simulink model "sm_pick_and_place_robot"  (R2021b)
settings: Solver=ode3  StartTime=0.0  StopTime=1.5  FixedStep=dt_solver  RelTol=1e-3  AbsTol=1e-3
model workspace (MAT data in the model file):
  dt_planner = 0.001
  dt_solver = 0.0002
undefined symbols (not defined in the file or in its folder): DiscIntNeverNeededParam, entire, Marker1, Marker2, Marker3, Marker4, point1, point2, point3, X, Y, Z
libraries: sm_lib x32, nesl_utility x17, sm_delta_robot_lib x1
(part 1 of 2)
CloseFcn:
  | clear sm_pick_and_place_robot_ik
  | clear sm_pick_and_place_robot_fk
Description:
  | Pick and Place Robot with Forward and Inverse Kinematics
settings Model: Creator=The MathWorks, Inc.  LastModifiedBy=The MathWorks, Inc.
settings SolverCC: AlgebraicLoopSolver=TrustRegion
settings DataIOCC: ReturnWorkspaceOutputs=off
settings DebuggingCC: SFMachineParentedDataDiag=warning
settings SimscapeCC: SimscapeLogType=all  SimscapeLogSimulationStatistics=on  SimscapeLogName=simlog_sm_pick_and_place_robot  SimscapeLogDataHistory=10000
settings ExplorerConfigSet: InternalSimMechanicsExplorerSettings="<ExplorerConfiguration><canonicalview>default</canonicalview><AnimationSetting><BasePlaybackSpeed>1.0</BasePlaybackSpeed><PlaybackSpeedFactor>1.0</PlaybackSpeedFactor></AnimationSetting><TilePanel><TileInfo><Tiles Columns=\"2\" Count=\"3\" Rows=\"2\"><Column Weight=\"0.5\"/><Column Weight=\"0.5\"/><Row Weight=\"0.3038\"/><Row Weight=\"0.6962\"/><Tile Height=\"2\" Width=\"1\" X=\"0\" Y=\"0\"/><Tile Height=\"1\" Width=\"1\" X=\"1\" Y=\"0\"/><Tile Height=\"1\" Width=\"1\" X=\"1\" Y=\"1\"/></Tiles></TileInfo><SceneInfo><SceneViewer><BGColor><R>0.60000002384185791</R><G>0.60000002384185791</G><B>0.60000002384185791</B></BGColor><Camera><DoPerspective>off</DoPerspective><Position><X>0.674555883500480347</X><Y>-0.674555883500480902</Y><Z>0.921885249943208973</Z></Position><Center><X>0.0060149771328419227</X><Y>-0.00601497713284246394</Y><Z>0.253344343575570674</Z></Center><Up><X>-0.408248290463863073</X><Y>0.408248290463863073</Y><Z>0.816496580927726145</Z></Up><ViewLimDist>1</ViewLimDist><YLim>0.43506960332393646</YLim><XLim>0.392966093324845833</XLim></Camera></SceneViewer><SceneViewer><BGColor><R>0.60000002384185791</R><G>0.60000002384185791</G><B>0.60000002384185791</B></BGColor><Camera><DoPerspective>off</DoPerspective><Position><X>-0.000385309004919674389</X><Y>-1.33915517216324798</Y><Z>0.0518624305243804845</Z></Position><Center><X>-0.000385309004919674389</X><Y>0.0454699993133544367</Y><Z>0.0518624305243804845</Z></Center><Up><X>0</X><Y>-0</Y><Z>1</Z></Up><ViewLimDist>1</ViewLimDist><YLim>0.0894075615531887413</YLim><XLim>0.282074560393158813</XLim></Camera></SceneViewer><SceneViewer><BGColor><R>0.60000002384185791</R><G>0.60000002384185791</G><B>0.60000002384185791</B></BGColor><Camera><DoPerspective>on</DoPerspective><Position><X>-1.13755508710961844e-18</X><Y>-8.63362207815730793e-18</Y><Z>0.589999999999999969</Z></Position><Center><X>-1.13755508710961844e-18</X><Y>-8.63362207815730793e-18</Y><Z>-0.410000000000000031</Z></Center><Up><X>0</X><Y>1</Y><Z>0</Z></Up><ViewLimDist>1</ViewLimDist><YLim>0.466307658154998583</YLim><XLim>0.621743544206664778</XLim></Camera></SceneViewer></SceneInfo></TilePanel><MechEditorPanel><Cameras><Camera><Id>Camera1</Id><Value><Name>CameraView</Name><NativeCamera><PositionTrackingFeature>Delta_Robot.Camera_Frame</PositionTrackingFeature><CenterTrackingFeature>Delta_Robot.Camera_Frame</CenterTrackingFeature><UpVectorTrackingFeature>Delta_Robot.Camera_Frame</UpVectorTrackingFeature><CenterTrackingOrigin>off</CenterTrackingOrigin><CenterTrackingDirection>+Z</CenterTrackingDirection><UpVectorTrackingDirection>-Y</UpVectorTrackingDirection></NativeCamera></Value></Camera></Cameras><GfxPanelCameraMap><MapElement CameraMLId=\"Camera1\" GfxPanelIndex=\"2\"/></GfxPanelCameraMap><VideoCreator><PlaybackSpeedRatio>1.0</PlaybackSpeedRatio><FrameRate>30</FrameRate><VideoFormat>Motion JPEG AVI</VideoFormat><FrameSize>auto</FrameSize></VideoCreator></MechEditorPanel></ExplorerConfiguration>"

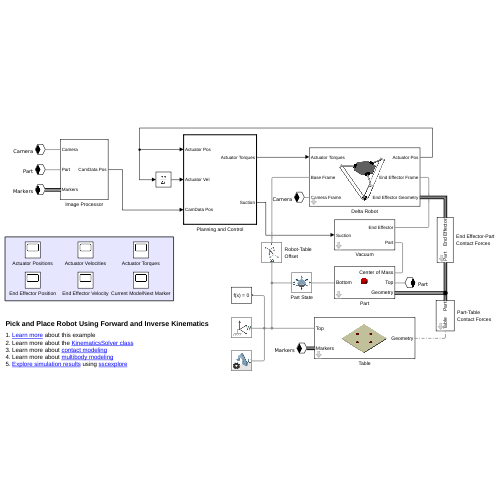
[thumbnail: Simulink's stored preview of the top-level diagram]
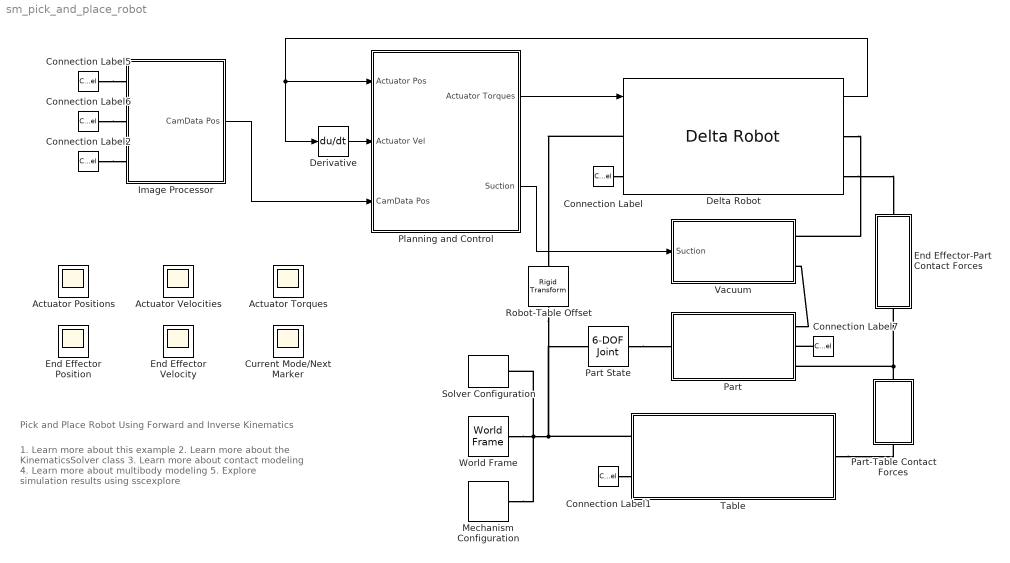
== system sm_pick_and_place_robot ==
  note: Pick and Place Robot Using Forward and Inverse Kinematics
  note: 1. Learn more about this example
      | 2. Learn more about the KinematicsSolver class
      | 3. Learn more about contact modeling
      | 4. Learn more about multibody modeling
      | 5. Explore simulation results using sscexplore
  Actuator Positions : Scope
      settings: Floating=on
  Actuator Torques : Scope
      settings: Floating=on
  Actuator Velocities : Scope
      settings: Floating=on
  Connection Label : ConnectionLabel  Label=Camera
  Connection Label1 : ConnectionLabel  Label=Markers
  Connection Label2 : ConnectionLabel  Label=Markers
  Connection Label5 : ConnectionLabel  Label=Camera
  Connection Label6 : ConnectionLabel  Label=Part
  Connection Label7 : ConnectionLabel  Label=Part
  Current Mode/Next Marker : Scope
      settings: Floating=on
  Delta Robot : sm_delta_robot_lib/Delta Robot  Rtop=0.15  Rbot=0.03  L1=0.2  R1=0.01  L2=0.5  L3=0.07  R2=0.005  eeL=0.03  eeR=0.01  th0=[10; 10; 10]  thd0=[0 0 0]  mask(Delta Robot){}
      mask init:
      | clear delta_robot_kf delta_robot_ik
      settings: SourceProductBaseCode=MS
  Derivative : Derivative  CoefficientInTFapproximation=dt_planner
  End Effector Position : Scope
      settings: Floating=on
  End Effector Velocity : Scope
      settings: Floating=on
  End Effector-Part Contact Forces : Subsystem  mask(End Effector-Part Contact Forces){k=1e6, b=10, mus=0.4, muk=0.4}
      mask prompts: k "Stiffness (N/m)"; b "Damping (N/(m/s))"; mus "Coefficient of Static Friction"; muk "Coefficient of Dynamic Friction"
      mask help: This block models the contact forces between the end effector and the part. The entire cylindrical part geometry is used, but the end effector geometry corresponds to the three contact points around the tip.
  Image Processor : Subsystem
  Mechanism Configuration : sm_lib/Utilities/Mechanism Configuration  UniformGravity=Constant  GravityVector=[0 0 -9.80665]  GravityUnits=m/s^2  LinearizationDelta=0.001  JointModeTransitionNonlinearIterations=2
  Part : Subsystem  mask(Part){R=0.02, H=0.02}
      mask prompts: R "Radius (m)"; H "Height (m)"
      mask help: This block models a cylindrical part. Frames at the center of the bottom face, center of the top face, and center of mass are exposed as ports. A Simscape Bus with geometry signals is also exposed. The bus includes the geometry of the entire part as well as the geometries of three evenly spaced points located around the edge of the bottom face of the cylinder.
      mask DialogControl ParameterGroupVar Prompt: Geometry
      mask Display: image(fullfile(matlabroot,'toolbox','physmod','sm','smdemos','pick_and_place_robot','images','sm_pick_and_place_robot_part.png'));
  Part State : sm_lib/Joints/6-DOF Joint  JointMode=Normal  SenseConstraintForce=off  SenseConstraintForceX=off  SenseConstraintForceY=off  SenseConstraintForceZ=off  SenseConstraintTorque=off  SenseConstraintTorqueX=off  SenseConstraintTorqueY=off  SenseConstraintTorqueZ=off  SenseTotalForce=off  SenseTotalForceX=off  SenseTotalForceY=off  SenseTotalForceZ=off  SenseTotalTorque=off  SenseTotalTorqueX=off  SenseTotalTorqueY=off  SenseTotalTorqueZ=off  CompositeWrenchDir=FollowerOnBase  CompositeWrenchFrame=BaseFrame  PxEquilibriumPosition=0  PxEquilibriumPositionUnits=m  PxSpringStiffness=0  PxSpringStiffnessUnits=N/m  PxDampingCoefficient=0  PxDampingCoefficientUnits=N/(m/s)  PxTorqueActuationMode=NoTorque  PxMotionActuationMode=ComputedMotion  PxSensePosition=off  PxSenseVelocity=off  PxSenseAcceleration=off  PxSenseTorqueForce=off  PxSenseLowerLimitTorqueForce=off  PxSenseUpperLimitTorqueForce=off  PxLowerLimitSpecify=off  PxLowerLimitBound=-1  PxLowerLimitBoundUnits=m  PxLowerLimitStiffness=1e6  PxLowerLimitStiffnessUnits=N/m  PxLowerLimitDamping=1e3  PxLowerLimitDampingUnits=N/(m/s)  PxLowerLimitTransitionRegionWidth=1e-4  PxLowerLimitTransitionRegionWidthUnits=m  PxUpperLimitSpecify=off  PxUpperLimitBound=1  PxUpperLimitBoundUnits=m  PxUpperLimitStiffness=1e6  PxUpperLimitStiffnessUnits=N/m  PxUpperLimitDamping=1e3  PxUpperLimitDampingUnits=N/(m/s)  PxUpperLimitTransitionRegionWidth=1e-4  PxUpperLimitTransitionRegionWidthUnits=m  PxPositionTargetSpecify=off  PxPositionTargetPriority=High  PxPositionTargetValue=0  PxPositionTargetValueUnits=m  PxVelocityTargetSpecify=off  PxVelocityTargetPriority=High  PxVelocityTargetValue=0  PxVelocityTargetValueUnits=m/s  PyEquilibriumPosition=0  PyEquilibriumPositionUnits=m  PySpringStiffness=0  PySpringStiffnessUnits=N/m  PyDampingCoefficient=0  PyDampingCoefficientUnits=N/(m/s)  PyTorqueActuationMode=NoTorque  PyMotionActuationMode=ComputedMotion  PySensePosition=off  PySenseVelocity=off  PySenseAcceleration=off  PySenseTorqueForce=off  PySenseLowerLimitTorqueForce=off  PySenseUpperLimitTorqueForce=off  PyLowerLimitSpecify=off  PyLowerLimitBound=-1  PyLowerLimitBoundUnits=m  PyLowerLimitStiffness=1e6  PyLowerLimitStiffnessUnits=N/m  PyLowerLimitDamping=1e3  PyLowerLimitDampingUnits=N/(m/s)  PyLowerLimitTransitionRegionWidth=1e-4  PyLowerLimitTransitionRegionWidthUnits=m  PyUpperLimitSpecify=off  PyUpperLimitBound=1  PyUpperLimitBoundUnits=m  PyUpperLimitStiffness=1e6  PyUpperLimitStiffnessUnits=N/m  PyUpperLimitDamping=1e3  PyUpperLimitDampingUnits=N/(m/s)  PyUpperLimitTransitionRegionWidth=1e-4  PyUpperLimitTransitionRegionWidthUnits=m  PyPositionTargetSpecify=off  PyPositionTargetPriority=High  PyPositionTargetValue=0  PyPositionTargetValueUnits=m  PyVelocityTargetSpecify=off  PyVelocityTargetPriority=High  PyVelocityTargetValue=0  PyVelocityTargetValueUnits=m/s  PzEquilibriumPosition=0  PzEquilibriumPositionUnits=m  PzSpringStiffness=0  PzSpringStiffnessUnits=N/m  PzDampingCoefficient=0  PzDampingCoefficientUnits=N/(m/s)  PzTorqueActuationMode=NoTorque  PzMotionActuationMode=ComputedMotion  PzSensePosition=off  PzSenseVelocity=off  PzSenseAcceleration=off  PzSenseTorqueForce=off  PzSenseLowerLimitTorqueForce=off  PzSenseUpperLimitTorqueForce=off  PzLowerLimitSpecify=off  PzLowerLimitBound=-1  PzLowerLimitBoundUnits=m  PzLowerLimitStiffness=1e6  PzLowerLimitStiffnessUnits=N/m  PzLowerLimitDamping=1e3  PzLowerLimitDampingUnits=N/(m/s)  PzLowerLimitTransitionRegionWidth=1e-4  PzLowerLimitTransitionRegionWidthUnits=m  PzUpperLimitSpecify=off  PzUpperLimitBound=1  PzUpperLimitBoundUnits=m  PzUpperLimitStiffness=1e6  PzUpperLimitStiffnessUnits=N/m  PzUpperLimitDamping=1e3  PzUpperLimitDampingUnits=N/(m/s)  PzUpperLimitTransitionRegionWidth=1e-4  PzUpperLimitTransitionRegionWidthUnits=m  PzPositionTargetSpecify=on  PzPositionTargetPriority=High  PzPositionTargetValue=0  PzPositionTargetValueUnits=m  PzVelocityTargetSpecify=off  PzVelocityTargetPriority=High  PzVelocityTargetValue=0  PzVelocityTargetValueUnits=m/s  SphDefPosRotationMethod=None  SphDefPosRotationAngleUnits=deg  SphDefPosRotationStandardAxis=+Z  SphDefPosRotationAngle=0.0  SphDefPosRotationArbitraryAxis=[0 0 1]  SphDefPosFollAlignAxisA=+X  SphDefPosBaseAlignAxisA=+Y  SphDefPosFollAlignAxisB=+Y  SphDefPosBaseAlignAxisB=+Z  SphDefPosRotationSequenceAxes=FollowerAxes  SphDefPosRotationSequence=XYX  SphDefPosRotationSequenceAngles=[0 0 0]  SphDefPosRotationSequenceAnglesUnits=deg  SphDefPosRotationMatrix=[1 0 0; 0 1 0; 0 0 1]  SphEqPosRotationMethod=None  SphEqPosRotationAngleUnits=deg  SphEqPosRotationStandardAxis=+Z  SphEqPosRotationAngle=0.0  SphEqPosRotationArbitraryAxis=[0 0 1]  SphEqPosFollAlignAxisA=+X  SphEqPosBaseAlignAxisA=+Y  SphEqPosFollAlignAxisB=+Y  SphEqPosBaseAlignAxisB=+Z  SphEqPosRotationSequenceAxes=FollowerAxes  SphEqPosRotationSequence=XYX  SphEqPosRotationSequenceAngles=[0 0 0]  SphEqPosRotationSequenceAnglesUnits=deg  SphEqPosRotationMatrix=[1 0 0; 0 1 0; 0 0 1]  SphSpringStiffness=0  SphSpringStiffnessUnits=N*m/deg  SphDampingCoefficient=0  SphDampingCoefficientUnits=N*m/(deg/s)  SphActuateTorqueX=off  SphActuateTorqueY=off  SphActuateTorqueZ=off  SphActuateTorque=off  SphTorqueActuationMode=NoTorque  SphMotionActuationMode=ComputedMotion  SphActuationFrame=BaseFrame  SphSensePosition=off  SphSenseVelocityX=off  SphSenseVelocityY=off  SphSenseVelocityZ=off  SphSenseVelocity=off  SphSenseAccelerationX=off  SphSenseAccelerationY=off  SphSenseAccelerationZ=off  SphSenseAcceleration=off  SphSenseTorqueX=off  SphSenseTorqueY=off  SphSenseTorqueZ=off  SphSenseTorqueForce=off  SphSenseLowerLimitTorqueMag=off  SphSenseUpperLimitTorqueMag=off  SphSensingFrame=BaseFrame  SphLowerLimitSpecify=off  SphLowerLimitBound=15  SphLowerLimitBoundUnits=deg  SphLowerLimitStiffness=1e4  SphLowerLimitStiffnessUnits=N*m/deg  SphLowerLimitDamping=10  SphLowerLimitDampingUnits=N*m/(deg/s)  SphLowerLimitTransitionRegionWidth=0.1  SphLowerLimitTransitionRegionWidthUnits=deg  SphUpperLimitSpecify=off  SphUpperLimitBound=45  SphUpperLimitBoundUnits=deg  SphUpperLimitStiffness=1e4  SphUpperLimitStiffnessUnits=N*m/deg  SphUpperLimitDamping=10  SphUpperLimitDampingUnits=N*m/(deg/s)  SphUpperLimitTransitionRegionWidth=0.1  SphUpperLimitTransitionRegionWidthUnits=deg  SphPositionTargetRotationMethod=None  SphPositionTargetRotationAngleUnits=deg  SphPositionTargetRotationStandardAxis=+Z  SphPositionTargetRotationAngle=0.0  SphPositionTargetRotationArbitraryAxis=[0 0 1]  SphPositionTargetFollAlignAxisA=+X  SphPositionTargetBaseAlignAxisA=+Y  SphPositionTargetFollAlignAxisB=+Y  SphPositionTargetBaseAlignAxisB=+Z  SphPositionTargetRotationSequenceAxes=FollowerAxes  SphPositionTargetRotationSequence=XYX  SphPositionTargetRotationSequenceAngles=[0 0 0]  SphPositionTargetRotationSequenceAnglesUnits=deg  SphPositionTargetRotationMatrix=[1 0 0; 0 1 0; 0 0 1]  SphPositionTargetSpecify=off  SphPositionTargetPriority=High  SphVelocityTargetValue=[0 0 0]  SphVelocityTargetValueUnits=deg/s  SphVelocityTargetSpecify=off  SphVelocityTargetPriority=High  SphVelocityTargetInFollowerFrame=on
  Part-Table Contact Forces : Subsystem  mask(Part-Base  Contact Forces){k=1e3, b=1e2, mus=0.3, muk=0.5}
      mask prompts: k "Stiffness (N/m)"; b "Damping (N/(m/s))"; mus "Coefficient of Static Friction"; muk "Coefficient of Dynamic Friction"
      mask help: This block models the contact forces between the partand the base platform. The part geometry corresponds to the three contact points on the bottom surface.
      settings: PortSchema="{\"entries\":[{\"content\":{\"sides\":[{\"content\":{\"connectorIds\":[]},\"type\":\"ConnectorPlacement.EquallySpacedRectSide\",\"uuid\":\"3ae6bdc3-8f46-45e0-9265-990a45186831\"},{\"content\":{\"connectorIds\":[],\"side\":\"RIGHT\"},\"type\":\"ConnectorPlacement.EquallySpacedRectSide\",\"uuid\":\"89855efe-6138-4444-8eb8-9815a715b27f\"},{\"content\":{\"connectorIds\":[\"LConn1\"],\"side\":\"TOP\"},\"type\":\"ConnectorPlacement.EquallySpacedRectSide\",\"uuid\":\"7a90f867-911e-4ba0-b8e7-edada11201ba\"},{\"content\":{\"connectorIds\":[\"RConn1\"],\"side\":\"BOTTOM\"},\"type\":\"ConnectorPlacement.EquallySpacedRectSide\",\"uuid\":\"8692366e-6cae-41d5-838e-6806be5f93d8\"}]},\"type\":\"ConnectorPlacement.EquallySpacedConnector\",\"uuid\":\"0998f4bf-2a7d-4302-bf06-c437b87cbd03\"}],\"packageUris\":[\"http://schema.mathworks.com/mf0/Connector/19700101\"],\"version\":\"1.0\"}"
  Planning and Control : Subsystem  TreatAsAtomicUnit=on  SystemSampleTime=dt_planner
  Robot-Table Offset : sm_lib/Frames and Transforms/Rigid Transform  TranslationMethod=StandardAxis  TranslationStandardOffset=0.6  TranslationLengthUnit=m  TranslationStandardAxis=+Z  TranslationCartesianOffset=[0 0 0]  TranslationROffset=0  TranslationROffsetUnits=m  TranslationZOffset=0  TranslationZOffsetUnits=m  TranslationThetaOffset=0  TranslationThetaOffsetUnits=deg  RotationMethod=None  RotationAngleUnits=deg  RotationStandardAxis=+Z  RotationAngle=0.0  RotationArbitraryAxis=[0 0 1]  FollAlignAxisA=+Z  BaseAlignAxisA=-Z  FollAlignAxisB=+X  BaseAlignAxisB=+X  RotationSequenceAxes=FollowerAxes  RotationSequence=XYX  RotationSequenceAngles=[0 0 0]  RotationSequenceAnglesUnits=deg  RotationMatrix=[1 0 0; 0 1 0; 0 0 1]
  Solver Configuration : nesl_utility/Solver Configuration  PhysicalDomain=network_engine_domain  SubClassName=solver  LeftPortType=input  RightPortType=generic  Tones=[]  Harmonics=[]  SimulateNoise=off  Profile=off  UseLocalSampling=off  EnableSwitchedLinearOptims=on  FrequencyDomain=off  UseCCode=off  RelTol=0.001  AbsTol=1e-06  MinStep=1e-09  ToWorkspace=off  RevertToSquareIcSolve=off  NumHomotopyIterations=100  PhasorMode=off  PhasorModeNumHarmonics=1  DoDC=off  ResidualTolerance=1e-09  UseLocalSolver=off  LocalSolverChoice=NE_BACKWARD_EULER_ADVANCER  LocalSolverSampleTime=0.001  DoFixedCost=off  MaxNonlinIter=3  MaxModeIter=2  ComputeImpulses=off  ImpulseIterations=2  LinearAlgebra=Sparse  EquationFormulation=NE_TIME_EF  DelaysMemoryBudget=1024  AutomaticFiltering=on  FilteringTimeConstant=0.001  PartitionStorageMethod=AS_NEEDED  PartitionMemoryBudget=1024  PartitionMethod=FAST
      settings: SourceProductBaseCode=PW,SS
  Table : Subsystem  mask(Base){L=0.5, H=0.02, d=0.15, clr=[1 1 0.8], r=0.025, mClr=[0.5 0 0]}
      mask prompts: L "Side Length (m)"; H "Height (m)"; d "Marker Distance From Center (m)"; clr "Color [R G B]"; r "Marker Radius (m)"; mClr "Marker Color [R G B]"
      mask help: Table with four equally spaced markers representing locations where a part can be placed by the robot.
      mask Display: image(fullfile(matlabroot,'toolbox','physmod','sm','smdemos','pick_and_place_robot','images','sm_pick_and_place_robot_base.png'));
  Vacuum : Subsystem  mask(Vacuum){F=20}
      mask prompts: F "Suction Force (N)"
      mask help: This block models a simple vacuum force in which equal and opposite constant forces are applied to two frames along the line connecting their origins. The force is only applied when the Suction signal is true.
  World Frame : sm_lib/Frames and Transforms/World Frame
  wires:
  Delta Robot/1 -> Planning and Control/1(Actuator Pos), Derivative/1
  Planning and Control/2(Suction) -> Vacuum/1(Suction)
  Image Processor/1(CamData Pos) -> Planning and Control/3(CamData Pos)
  Derivative/1 -> Planning and Control/2(Actuator Vel)
  Planning and Control/1(Actuator Torques) -> Delta Robot/1
  connections:
  Connection Label/LConn1 -- Delta Robot/LConn2
  Part/RConn1 -- Vacuum/RConn2
  Part-Table Contact Forces/LConn1 -- End Effector-Part Contact Forces/RConn1 -- Part/RConn3
  Table/RConn1 -- Part-Table Contact Forces/RConn1
  Connection Label5/LConn1 -- Image Processor/LConn1
  Connection Label6/LConn1 -- Image Processor/LConn2
  Delta Robot/RConn1 -- Vacuum/RConn1
  Connection Label7/LConn1 -- Part/RConn2
  Delta Robot/RConn2 -- End Effector-Part Contact Forces/LConn1
  World Frame/RConn1 -- Solver Configuration/RConn1 -- Table/LConn1 -- Robot-Table Offset/LConn1 -- Part State/LConn1 -- Mechanism Configuration/RConn1
  Connection Label1/LConn1 -- Table/LConn2
  Connection Label2/LConn1 -- Image Processor/LConn3
  Part State/RConn1 -- Part/LConn1
  Delta Robot/LConn1 -- Robot-Table Offset/RConn1

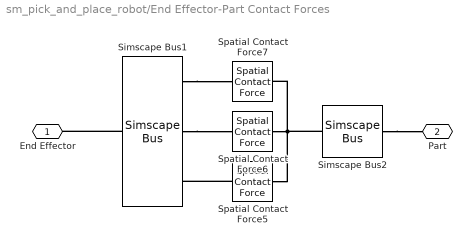
== system sm_pick_and_place_robot/End Effector-Part Contact Forces ==
  Simscape Bus1 : SimscapeBus  HierarchyStrings=point1;point2;point3
  Simscape Bus2 : SimscapeBus  HierarchyStrings=entire
  Spatial Contact Force5 : sm_lib/Forces and Torques/Spatial Contact Force  CoefficientOfDynamicFriction=muk  CoefficientOfStaticFriction=mus  SenseContactBaseRotation=off  SenseContactBaseTranslation=off  NormalDamping=b  NormalDampingUnits=N/(m/s)  SenseContactFollowerRotation=off  SenseContactFollowerTranslation=off  SenseContactSignal=off  NormalStiffness=k  NormalStiffnessUnits=N/m  FrictionalCriticalVelocity=1e-3  FrictionalCriticalVelocityUnits=m/s  ZeroCrossDetectContactStartAndEnd=off  FrictionType=SmoothStickSlip  SenseFrictionalForceMagnitude=off  SenseNormalForceMagnitude=off  NormalForceType=SmoothSpringDamper  SenseNormalVelocity=off  SenseSeparationDistance=off  SenseTangentialVelocity=off  SenseTangentialVelocityMagnitude=off  NormalTransitionRegionWidth=1e-4  NormalTransitionRegionWidthUnits=m
  Spatial Contact Force6 : sm_lib/Forces and Torques/Spatial Contact Force  CoefficientOfDynamicFriction=muk  CoefficientOfStaticFriction=mus  SenseContactBaseRotation=off  SenseContactBaseTranslation=off  NormalDamping=b  NormalDampingUnits=N/(m/s)  SenseContactFollowerRotation=off  SenseContactFollowerTranslation=off  SenseContactSignal=off  NormalStiffness=k  NormalStiffnessUnits=N/m  FrictionalCriticalVelocity=1e-3  FrictionalCriticalVelocityUnits=m/s  ZeroCrossDetectContactStartAndEnd=off  FrictionType=SmoothStickSlip  SenseFrictionalForceMagnitude=off  SenseNormalForceMagnitude=off  NormalForceType=SmoothSpringDamper  SenseNormalVelocity=off  SenseSeparationDistance=off  SenseTangentialVelocity=off  SenseTangentialVelocityMagnitude=off  NormalTransitionRegionWidth=1e-4  NormalTransitionRegionWidthUnits=m
  Spatial Contact Force7 : sm_lib/Forces and Torques/Spatial Contact Force  CoefficientOfDynamicFriction=muk  CoefficientOfStaticFriction=mus  SenseContactBaseRotation=off  SenseContactBaseTranslation=off  NormalDamping=b  NormalDampingUnits=N/(m/s)  SenseContactFollowerRotation=off  SenseContactFollowerTranslation=off  SenseContactSignal=off  NormalStiffness=k  NormalStiffnessUnits=N/m  FrictionalCriticalVelocity=1e-3  FrictionalCriticalVelocityUnits=m/s  ZeroCrossDetectContactStartAndEnd=off  FrictionType=SmoothStickSlip  SenseFrictionalForceMagnitude=off  SenseNormalForceMagnitude=off  NormalForceType=SmoothSpringDamper  SenseNormalVelocity=off  SenseSeparationDistance=off  SenseTangentialVelocity=off  SenseTangentialVelocityMagnitude=off  NormalTransitionRegionWidth=1e-4  NormalTransitionRegionWidthUnits=m
  End Effector : PMIOPort  Side=Left
  Part : PMIOPort  Port=2  Side=Right
  connections:
  Simscape Bus1/LConn1 -- Spatial Contact Force7/LConn1
  Spatial Contact Force5/LConn1 -- Simscape Bus1/LConn3
  Spatial Contact Force6/RConn1 -- Simscape Bus2/LConn1 -- Spatial Contact Force5/RConn1 -- Spatial Contact Force7/RConn1
  Simscape Bus1/LConn2 -- Spatial Contact Force6/LConn1
  Simscape Bus1/RConn1 -- End Effector/RConn1
  Simscape Bus2/RConn1 -- Part/RConn1

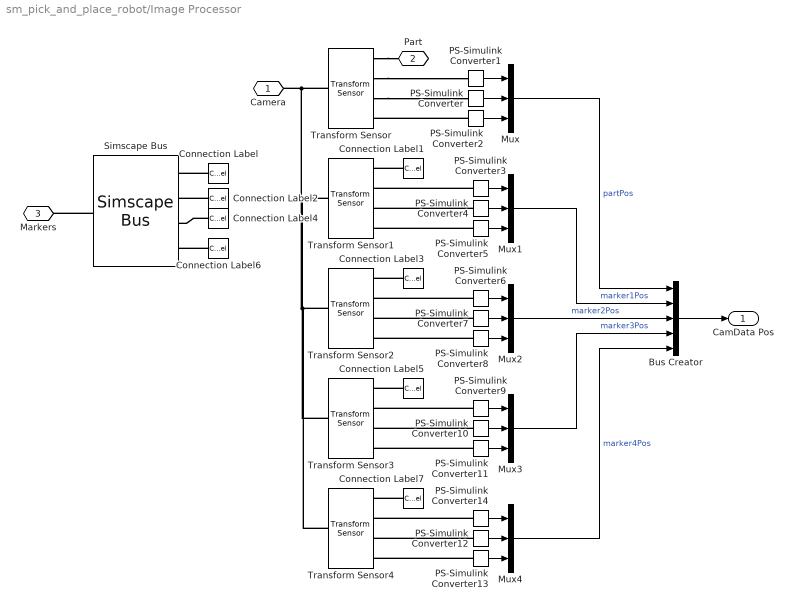
== system sm_pick_and_place_robot/Image Processor ==
  Bus Creator : BusCreator  Inputs=5
  Connection Label : ConnectionLabel  Label=Marker1
  Connection Label1 : ConnectionLabel  Label=Marker1
  Connection Label2 : ConnectionLabel  Label=Marker2
  Connection Label3 : ConnectionLabel  Label=Marker2
  Connection Label4 : ConnectionLabel  Label=Marker3
  Connection Label5 : ConnectionLabel  Label=Marker3
  Connection Label6 : ConnectionLabel  Label=Marker4
  Connection Label7 : ConnectionLabel  Label=Marker4
  Mux{,1..4} (5 alike) : Mux  Inputs=3
  PS-Simulink Converter{,1..14} (15 alike) : nesl_utility/PS-Simulink Converter  PhysicalDomain=network_engine_domain  SubClassName=ps_output  LeftPortType=input  RightPortType=output  PseudoPeriodic=off  Frequencies=[]  Unit=m  AffineConversion=off
      settings: SourceProductBaseCode=PW,SS
  Simscape Bus : SimscapeBus  HierarchyStrings=Marker1;Marker2;Marker3;Marker4
  Transform Sensor{,1..4} (5 alike) : sm_lib/Frames and Transforms/Transform Sensor  MeasurementFrame=Base  SenseAngle=off  SenseAxis=off  SenseAngle1=off  SenseAngle2=off  SenseAngle3=off  SenseQ=off  SenseR=off  SenseOmegaX=off  SenseOmegaY=off  SenseOmegaZ=off  SenseOmega1=off  SenseOmega2=off  SenseOmega3=off  SenseQDot=off  SenseRDot=off  SenseAlphaX=off  SenseAlphaY=off  SenseAlphaZ=off  SenseAlpha1=off  SenseAlpha2=off  SenseAlpha3=off  SenseQDDot=off  SenseRDDot=off  SenseX=on  SenseY=on  SenseZ=on  SenseRad=off  SenseAzim=off  SenseDist=off  SenseInc=off  SenseXDot=off  SenseYDot=off  SenseZDot=off  SenseRadDot=off  SenseAzimDot=off  SenseDistDot=off  SenseIncDot=off  SenseXDDot=off  SenseYDDot=off  SenseZDDot=off  SenseRadDDot=off  SenseAzimDDot=off  SenseDistDDot=off  SenseIncDDot=off
  Camera : PMIOPort  Side=Left
  Part : PMIOPort  Port=2  Side=Left
  Markers : PMIOPort  Port=3  Side=Left
  CamData Pos : Outport
  wires:
  PS-Simulink Converter1/1 -> Mux/1
  PS-Simulink Converter/1 -> Mux/2
  PS-Simulink Converter2/1 -> Mux/3
  Mux/1 -> Bus Creator/1  "partPos"
  Mux1/1 -> Bus Creator/2  "marker1Pos"
  PS-Simulink Converter4/1 -> Mux1/2
  PS-Simulink Converter5/1 -> Mux1/3
  PS-Simulink Converter3/1 -> Mux1/1
  Mux2/1 -> Bus Creator/3  "marker2Pos"
  PS-Simulink Converter7/1 -> Mux2/2
  PS-Simulink Converter8/1 -> Mux2/3
  PS-Simulink Converter6/1 -> Mux2/1
  Bus Creator/1 -> CamData Pos/1
  Mux3/1 -> Bus Creator/4  "marker3Pos"
  PS-Simulink Converter11/1 -> Mux3/3
  PS-Simulink Converter9/1 -> Mux3/1
  PS-Simulink Converter10/1 -> Mux3/2
  Mux4/1 -> Bus Creator/5  "marker4Pos"
  PS-Simulink Converter12/1 -> Mux4/2
  PS-Simulink Converter14/1 -> Mux4/1
  PS-Simulink Converter13/1 -> Mux4/3
  connections:
  Transform Sensor/LConn1 -- Transform Sensor4/LConn1 -- Transform Sensor3/LConn1 -- Transform Sensor2/LConn1 -- Transform Sensor1/LConn1 -- Camera/RConn1
  Transform Sensor/RConn1 -- Part/RConn1
  Transform Sensor/RConn2 -- PS-Simulink Converter1/LConn1
  Transform Sensor/RConn3 -- PS-Simulink Converter/LConn1
  PS-Simulink Converter2/LConn1 -- Transform Sensor/RConn4
  Connection Label1/LConn1 -- Transform Sensor1/RConn1
  PS-Simulink Converter3/LConn1 -- Transform Sensor1/RConn2
  PS-Simulink Converter5/LConn1 -- Transform Sensor1/RConn4
  PS-Simulink Converter4/LConn1 -- Transform Sensor1/RConn3
  Connection Label3/LConn1 -- Transform Sensor2/RConn1
  PS-Simulink Converter6/LConn1 -- Transform Sensor2/RConn2
  PS-Simulink Converter8/LConn1 -- Transform Sensor2/RConn4
  PS-Simulink Converter7/LConn1 -- Transform Sensor2/RConn3
  Simscape Bus/RConn1 -- Markers/RConn1
  Connection Label5/LConn1 -- Transform Sensor3/RConn1
  PS-Simulink Converter11/LConn1 -- Transform Sensor3/RConn4
  PS-Simulink Converter9/LConn1 -- Transform Sensor3/RConn2
  PS-Simulink Converter10/LConn1 -- Transform Sensor3/RConn3
  PS-Simulink Converter14/LConn1 -- Transform Sensor4/RConn2
  Connection Label7/LConn1 -- Transform Sensor4/RConn1
  PS-Simulink Converter12/LConn1 -- Transform Sensor4/RConn3
  PS-Simulink Converter13/LConn1 -- Transform Sensor4/RConn4
  Connection Label/LConn1 -- Simscape Bus/LConn1
  Connection Label2/LConn1 -- Simscape Bus/LConn2
  Connection Label4/LConn1 -- Simscape Bus/LConn3
  Connection Label6/LConn1 -- Simscape Bus/LConn4

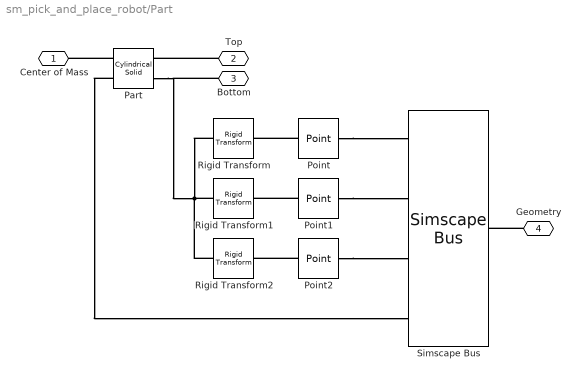
== system sm_pick_and_place_robot/Part ==
  Part : sm_lib/Body Elements/Cylindrical Solid  GraphicAmbientColor=[0.15 0.15 0.15 1.0]  BasedOnType=Density  CenterOfMass=[0 0 0]  CenterOfMassUnits=m  GraphicDiffuseColor=[1.0 0.0 0.0]  CylinderLength=H  CylinderLengthUnits=m  CylinderRadius=R  CylinderRadiusUnits=m  Density=1000  DensityUnits=kg/m^3  DoExposeReferenceFrame=on  GraphicEmissiveColor=[0.0 0.0 0.0 1.0]  ExportEntireGeometry=on  SerializedFrames=<Frames><Frame><Id>Frame1</Id><Value><Name>top</Name><Origin><Source>GeometricFeature</Source><FeatureName>top surface</FeatureName></Origin><PrimaryAxis><DefinedDirection>+Z</DefinedDirection><Source>ReferenceFrame</Source><SourceDirection>+Z</SourceDirection><FeatureName></FeatureName></PrimaryAxis><SecondaryAxis><DefinedDirection>+X</DefinedDirection><Source>ReferenceFrame</Source><SourceDirection>+X</SourceDirection><FeatureName></FeatureName></SecondaryAxis></Value></Frame><Frame><Id>Frame2</Id><Value><Name>bot</Name><Origin><Source>GeometricFeature</Source><FeatureName>bottom surface</FeatureName></Origin><PrimaryAxis><DefinedDirection>+Z</DefinedDirection><Source>ReferenceFrame</Source><SourceDirection>+Z</SourceDirection><FeatureName></FeatureName></PrimaryAxis><SecondaryAxis><DefinedDirection>+X</DefinedDirection><Source>ReferenceFrame</Source><SourceDirection>+X</SourceDirection><FeatureName></FeatureName></SecondaryAxis></Value></Frame></Frames>  MarkerShape=Sphere  MarkerSize=10  GraphicType=FromGeometry  InertiaType=CalculateFromGeometry  Mass=1  MassUnits=kg  MomentsOfInertia=[1 1 1]  MomentsOfInertiaUnits=kg*m^2  GraphicOpacity=1.0  ProductsOfInertia=[0 0 0]  ProductsOfInertiaUnits=kg*m^2  GraphicShininess=75  GraphicSpecularColor=[0.5 0.5 0.5 1.0]  GraphicVisPropType=SimpleVisualProperties
  Point : sm_lib/Curves and Surfaces/Point  GraphicType=None  MarkerShape=Sphere  MarkerSize=2  GraphicVisPropType=SimpleVisualProperties  GraphicDiffuseColor=[0.5 0.5 0.5]  GraphicOpacity=1.0  GraphicSpecularColor=[0.5 0.5 0.5 1.0]  GraphicAmbientColor=[0.15 0.15 0.15 1.0]  GraphicEmissiveColor=[0.0 0.0 0.0 1.0]  GraphicShininess=75
      settings: SourceProductBaseCode=MS
  Point1 : sm_lib/Curves and Surfaces/Point  GraphicType=None  MarkerShape=Sphere  MarkerSize=2  GraphicVisPropType=SimpleVisualProperties  GraphicDiffuseColor=[0.5 0.5 0.5]  GraphicOpacity=1.0  GraphicSpecularColor=[0.5 0.5 0.5 1.0]  GraphicAmbientColor=[0.15 0.15 0.15 1.0]  GraphicEmissiveColor=[0.0 0.0 0.0 1.0]  GraphicShininess=75
      settings: SourceProductBaseCode=MS
  Point2 : sm_lib/Curves and Surfaces/Point  GraphicType=None  MarkerShape=Sphere  MarkerSize=2  GraphicVisPropType=SimpleVisualProperties  GraphicDiffuseColor=[0.5 0.5 0.5]  GraphicOpacity=1.0  GraphicSpecularColor=[0.5 0.5 0.5 1.0]  GraphicAmbientColor=[0.15 0.15 0.15 1.0]  GraphicEmissiveColor=[0.0 0.0 0.0 1.0]  GraphicShininess=75
      settings: SourceProductBaseCode=MS
  Rigid Transform : sm_lib/Frames and Transforms/Rigid Transform  TranslationMethod=Cartesian  TranslationStandardOffset=R  TranslationLengthUnit=m  TranslationStandardAxis=+X  TranslationCartesianOffset=[R 0 0]  TranslationROffset=0  TranslationROffsetUnits=m  TranslationZOffset=0  TranslationZOffsetUnits=m  TranslationThetaOffset=0  TranslationThetaOffsetUnits=deg  RotationMethod=None  RotationAngleUnits=deg  RotationStandardAxis=+Z  RotationAngle=0.0  RotationArbitraryAxis=[0 0 1]  FollAlignAxisA=+X  BaseAlignAxisA=+Y  FollAlignAxisB=+Y  BaseAlignAxisB=+Z  RotationSequenceAxes=FollowerAxes  RotationSequence=XYX  RotationSequenceAngles=[0 0 0]  RotationSequenceAnglesUnits=deg  RotationMatrix=[1 0 0; 0 1 0; 0 0 1]
  Rigid Transform1 : sm_lib/Frames and Transforms/Rigid Transform  TranslationMethod=Cartesian  TranslationStandardOffset=R  TranslationLengthUnit=m  TranslationStandardAxis=+X  TranslationCartesianOffset=[R*cosd(120) R*sind(120) 0]  TranslationROffset=0  TranslationROffsetUnits=m  TranslationZOffset=0  TranslationZOffsetUnits=m  TranslationThetaOffset=0  TranslationThetaOffsetUnits=deg  RotationMethod=None  RotationAngleUnits=deg  RotationStandardAxis=+Z  RotationAngle=0  RotationArbitraryAxis=[0 0 1]  FollAlignAxisA=+X  BaseAlignAxisA=+Y  FollAlignAxisB=+Y  BaseAlignAxisB=+Z  RotationSequenceAxes=FollowerAxes  RotationSequence=XYX  RotationSequenceAngles=[0 0 0]  RotationSequenceAnglesUnits=deg  RotationMatrix=[1 0 0; 0 1 0; 0 0 1]
  Rigid Transform2 : sm_lib/Frames and Transforms/Rigid Transform  TranslationMethod=Cartesian  TranslationStandardOffset=R  TranslationLengthUnit=m  TranslationStandardAxis=+X  TranslationCartesianOffset=[R*cosd(240) R*sind(240) 0]  TranslationROffset=0  TranslationROffsetUnits=m  TranslationZOffset=0  TranslationZOffsetUnits=m  TranslationThetaOffset=0  TranslationThetaOffsetUnits=deg  RotationMethod=None  RotationAngleUnits=deg  RotationStandardAxis=+Z  RotationAngle=0  RotationArbitraryAxis=[0 0 1]  FollAlignAxisA=+X  BaseAlignAxisA=+Y  FollAlignAxisB=+Y  BaseAlignAxisB=+Z  RotationSequenceAxes=FollowerAxes  RotationSequence=XYX  RotationSequenceAngles=[0 0 0]  RotationSequenceAnglesUnits=deg  RotationMatrix=[1 0 0; 0 1 0; 0 0 1]
  Simscape Bus : SimscapeBus  HierarchyStrings=point1;point2;point3;entire
  Center of Mass : PMIOPort  Side=Right
  Top : PMIOPort  Port=2  Side=Right
  Bottom : PMIOPort  Port=3  Side=Left
  Geometry : PMIOPort  Port=4  Side=Right
  connections:
  Part/RConn1 -- Center of Mass/RConn1
  Top/RConn1 -- Part/LConn1
  Point/LConn1 -- Rigid Transform/RConn1
  Rigid Transform1/LConn1 -- Bottom/RConn1 -- Part/LConn2 -- Rigid Transform2/LConn1 -- Rigid Transform/LConn1
  Point1/LConn1 -- Rigid Transform1/RConn1
  Point2/LConn1 -- Rigid Transform2/RConn1
  Point1/RConn1 -- Simscape Bus/LConn2
  Point/RConn1 -- Simscape Bus/LConn1
  Point2/RConn1 -- Simscape Bus/LConn3
  Geometry/RConn1 -- Simscape Bus/RConn1
  Part/RConn2 -- Simscape Bus/LConn4

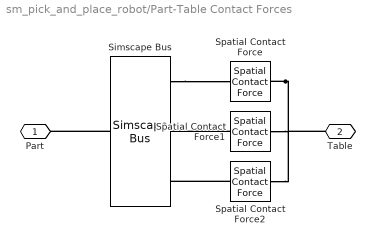
== system sm_pick_and_place_robot/Part-Table Contact Forces ==
  Simscape Bus : SimscapeBus  HierarchyStrings=point1;point2;point3
  Spatial Contact Force : sm_lib/Forces and Torques/Spatial Contact Force  CoefficientOfDynamicFriction=muk  CoefficientOfStaticFriction=mus  SenseContactBaseRotation=off  SenseContactBaseTranslation=off  NormalDamping=b  NormalDampingUnits=N/(m/s)  SenseContactFollowerRotation=off  SenseContactFollowerTranslation=off  SenseContactSignal=off  NormalStiffness=k  NormalStiffnessUnits=N/m  FrictionalCriticalVelocity=1e-3  FrictionalCriticalVelocityUnits=m/s  ZeroCrossDetectContactStartAndEnd=off  FrictionType=SmoothStickSlip  SenseFrictionalForceMagnitude=off  SenseNormalForceMagnitude=off  NormalForceType=SmoothSpringDamper  SenseNormalVelocity=off  SenseSeparationDistance=off  SenseTangentialVelocity=off  SenseTangentialVelocityMagnitude=off  NormalTransitionRegionWidth=1e-4  NormalTransitionRegionWidthUnits=m
  Spatial Contact Force1 : sm_lib/Forces and Torques/Spatial Contact Force  CoefficientOfDynamicFriction=muk  CoefficientOfStaticFriction=mus  SenseContactBaseRotation=off  SenseContactBaseTranslation=off  NormalDamping=b  NormalDampingUnits=N/(m/s)  SenseContactFollowerRotation=off  SenseContactFollowerTranslation=off  SenseContactSignal=off  NormalStiffness=k  NormalStiffnessUnits=N/m  FrictionalCriticalVelocity=1e-3  FrictionalCriticalVelocityUnits=m/s  ZeroCrossDetectContactStartAndEnd=off  FrictionType=SmoothStickSlip  SenseFrictionalForceMagnitude=off  SenseNormalForceMagnitude=off  NormalForceType=SmoothSpringDamper  SenseNormalVelocity=off  SenseSeparationDistance=off  SenseTangentialVelocity=off  SenseTangentialVelocityMagnitude=off  NormalTransitionRegionWidth=1e-4  NormalTransitionRegionWidthUnits=m
  Spatial Contact Force2 : sm_lib/Forces and Torques/Spatial Contact Force  CoefficientOfDynamicFriction=muk  CoefficientOfStaticFriction=mus  SenseContactBaseRotation=off  SenseContactBaseTranslation=off  NormalDamping=b  NormalDampingUnits=N/(m/s)  SenseContactFollowerRotation=off  SenseContactFollowerTranslation=off  SenseContactSignal=off  NormalStiffness=k  NormalStiffnessUnits=N/m  FrictionalCriticalVelocity=1e-3  FrictionalCriticalVelocityUnits=m/s  ZeroCrossDetectContactStartAndEnd=off  FrictionType=SmoothStickSlip  SenseFrictionalForceMagnitude=off  SenseNormalForceMagnitude=off  NormalForceType=SmoothSpringDamper  SenseNormalVelocity=off  SenseSeparationDistance=off  SenseTangentialVelocity=off  SenseTangentialVelocityMagnitude=off  NormalTransitionRegionWidth=1e-4  NormalTransitionRegionWidthUnits=m
  Part : PMIOPort  Side=Left
  Table : PMIOPort  Port=2  Side=Right
  connections:
  Simscape Bus/RConn1 -- Part/RConn1
  Simscape Bus/LConn1 -- Spatial Contact Force/LConn1
  Spatial Contact Force2/LConn1 -- Simscape Bus/LConn3
  Spatial Contact Force1/LConn1 -- Simscape Bus/LConn2
  Spatial Contact Force/RConn1 -- Table/RConn1 -- Spatial Contact Force2/RConn1 -- Spatial Contact Force1/RConn1

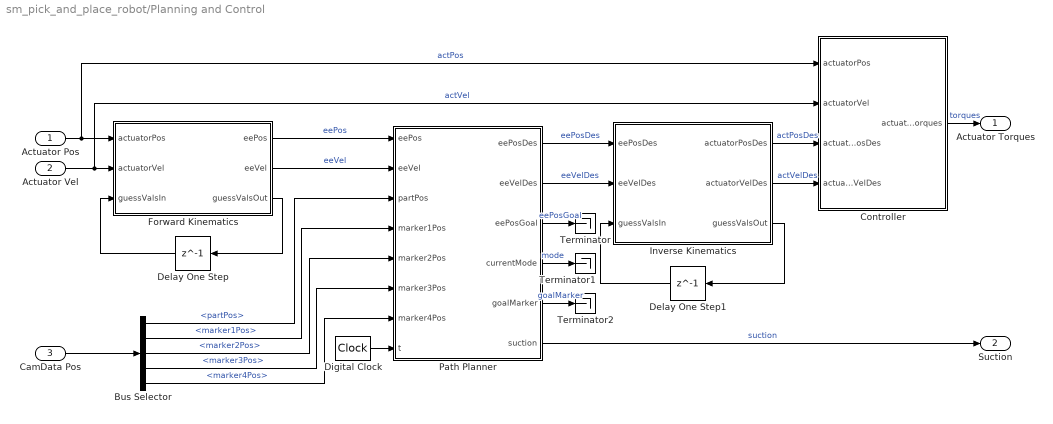
== system sm_pick_and_place_robot/Planning and Control ==
  Actuator Pos : Inport
  Actuator Vel : Inport  Port=2
  CamData Pos : Inport  Port=3
  Bus Selector : BusSelector  OutputSignals=partPos,marker1Pos,marker2Pos,marker3Pos,marker4Pos
  Controller : Subsystem  TreatAsAtomicUnit=on  mask(PID Controller){P=0.5, I=6, D=0.15}
  Delay One Step : Delay  DelayLength=1
  Delay One Step1 : Delay  DelayLength=1
  Digital Clock : DigitalClock  SampleTime=dt_planner
  Forward Kinematics : MATLAB Function  TreatAsAtomicUnit=on
  Inverse Kinematics : MATLAB Function  TreatAsAtomicUnit=on
  Path Planner : MATLAB Function  TreatAsAtomicUnit=on
  Terminator : Terminator
  Terminator1 : Terminator
  Terminator2 : Terminator
  Actuator Torques : Outport
  Suction : Outport  Port=2
  wires:
  Forward Kinematics/3(guessValsOut) -> Delay One Step/1
  Delay One Step/1 -> Forward Kinematics/3(guessValsIn)
  Inverse Kinematics/1(actuatorPosDes) -> Controller/3(actuatorPosDes)  "actPosDes"
  Forward Kinematics/1(eePos) -> Path Planner/1(eePos)  "eePos"
  Path Planner/1(eePosDes) -> Inverse Kinematics/1(eePosDes)  "eePosDes"
  Path Planner/6(suction) -> Suction/1  "suction"
  Inverse Kinematics/3(guessValsOut) -> Delay One Step1/1
  Delay One Step1/1 -> Inverse Kinematics/3(guessValsIn)
  Actuator Pos/1 -> Forward Kinematics/1(actuatorPos), Controller/1(actuatorPos)  "actPos"
  CamData Pos/1 -> Bus Selector/1
  Bus Selector/1 -> Path Planner/3(partPos)  "<partPos>"
  Bus Selector/2 -> Path Planner/4(marker1Pos)  "<marker1Pos>"
  Bus Selector/3 -> Path Planner/5(marker2Pos)  "<marker2Pos>"
  Digital Clock/1 -> Path Planner/8(t)
  Actuator Vel/1 -> Forward Kinematics/2(actuatorVel), Controller/2(actuatorVel)  "actVel"
  Forward Kinematics/2(eeVel) -> Path Planner/2(eeVel)  "eeVel"
  Path Planner/2(eeVelDes) -> Inverse Kinematics/2(eeVelDes)  "eeVelDes"
  Inverse Kinematics/2(actuatorVelDes) -> Controller/4(actuatorVelDes)  "actVelDes"
  Bus Selector/4 -> Path Planner/6(marker3Pos)  "<marker3Pos>"
  Bus Selector/5 -> Path Planner/7(marker4Pos)  "<marker4Pos>"
  Controller/1(actuatorTorques) -> Actuator Torques/1  "torques"
  Path Planner/3(eePosGoal) -> Terminator/1  "eePosGoal"
  Path Planner/4(currentMode) -> Terminator1/1  "mode"
  Path Planner/5(goalMarker) -> Terminator2/1  "goalMarker"

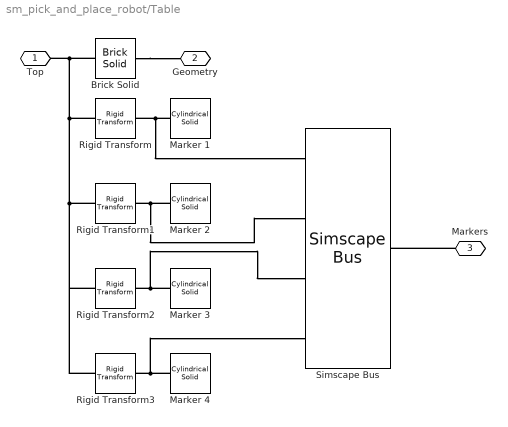
== system sm_pick_and_place_robot/Table ==
  Brick Solid : sm_lib/Body Elements/Brick Solid  GraphicAmbientColor=[0.15 0.15 0.15 1.0]  BasedOnType=Density  BrickDimensions=[L L H]  BrickDimensionUnits=m  CenterOfMass=[0 0 0]  CenterOfMassUnits=m  GraphicDiffuseColor=clr  Density=0  DensityUnits=kg/m^3  DoExposeReferenceFrame=off  GraphicEmissiveColor=[0.0 0.0 0.0 1.0]  ExportEntireGeometry=on  SerializedFrames=<Frames><Frame><Id>Frame1</Id><Value><Name>top</Name><Origin><Source>GeometricFeature</Source><FeatureName>+z surface</FeatureName></Origin><PrimaryAxis><DefinedDirection>+Z</DefinedDirection><Source>ReferenceFrame</Source><SourceDirection>+Z</SourceDirection><FeatureName></FeatureName></PrimaryAxis><SecondaryAxis><DefinedDirection>+X</DefinedDirection><Source>ReferenceFrame</Source><SourceDirection>+X</SourceDirection><FeatureName></FeatureName></SecondaryAxis></Value></Frame></Frames>  MarkerShape=Sphere  MarkerSize=10  GraphicType=FromGeometry  InertiaType=CalculateFromGeometry  Mass=1  MassUnits=kg  MomentsOfInertia=[1 1 1]  MomentsOfInertiaUnits=kg*m^2  GraphicOpacity=1.0  ProductsOfInertia=[0 0 0]  ProductsOfInertiaUnits=kg*m^2  GraphicShininess=75  GraphicSpecularColor=[0.5 0.5 0.5 1.0]  GraphicVisPropType=SimpleVisualProperties
  Marker {1..4} (4 alike) : sm_lib/Body Elements/Cylindrical Solid  GraphicAmbientColor=[0.15 0.15 0.15 1.0]  BasedOnType=Density  CenterOfMass=[0 0 0]  CenterOfMassUnits=m  GraphicDiffuseColor=mClr  CylinderLength=H/100  CylinderLengthUnits=m  CylinderRadius=r  CylinderRadiusUnits=m  Density=0  DensityUnits=kg/m^3  DoExposeReferenceFrame=off  GraphicEmissiveColor=[0.0 0.0 0.0 1.0]  ExportEntireGeometry=off  SerializedFrames=<Frames><Frame><Id>Frame1</Id><Value><Name>bot</Name><Origin><Source>GeometricFeature</Source><FeatureName>bottom surface</FeatureName></Origin><PrimaryAxis><DefinedDirection>+Z</DefinedDirection><Source>ReferenceFrame</Source><SourceDirection>+Z</SourceDirection><FeatureName></FeatureName></PrimaryAxis><SecondaryAxis><DefinedDirection>+X</DefinedDirection><Source>ReferenceFrame</Source><SourceDirection>+X</SourceDirection><FeatureName></FeatureName></SecondaryAxis></Value></Frame></Frames>  MarkerShape=Sphere  MarkerSize=10  GraphicType=FromGeometry  InertiaType=CalculateFromGeometry  Mass=1  MassUnits=kg  MomentsOfInertia=[1 1 1]  MomentsOfInertiaUnits=kg*m^2  GraphicOpacity=1.0  ProductsOfInertia=[0 0 0]  ProductsOfInertiaUnits=kg*m^2  GraphicShininess=75  GraphicSpecularColor=[0.5 0.5 0.5 1.0]  GraphicVisPropType=SimpleVisualProperties
  Rigid Transform : sm_lib/Frames and Transforms/Rigid Transform  TranslationMethod=Cartesian  TranslationStandardOffset=0  TranslationLengthUnit=m  TranslationStandardAxis=+Z  TranslationCartesianOffset=[d 0 0]  TranslationROffset=0  TranslationROffsetUnits=m  TranslationZOffset=0  TranslationZOffsetUnits=m  TranslationThetaOffset=0  TranslationThetaOffsetUnits=deg  RotationMethod=None  RotationAngleUnits=deg  RotationStandardAxis=+Z  RotationAngle=0.0  RotationArbitraryAxis=[0 0 1]  FollAlignAxisA=+X  BaseAlignAxisA=+Y  FollAlignAxisB=+Y  BaseAlignAxisB=+Z  RotationSequenceAxes=FollowerAxes  RotationSequence=XYX  RotationSequenceAngles=[0 0 0]  RotationSequenceAnglesUnits=deg  RotationMatrix=[1 0 0; 0 1 0; 0 0 1]
  Rigid Transform1 : sm_lib/Frames and Transforms/Rigid Transform  TranslationMethod=Cartesian  TranslationStandardOffset=0  TranslationLengthUnit=m  TranslationStandardAxis=+Z  TranslationCartesianOffset=[0 d 0]  TranslationROffset=0  TranslationROffsetUnits=m  TranslationZOffset=0  TranslationZOffsetUnits=m  TranslationThetaOffset=0  TranslationThetaOffsetUnits=deg  RotationMethod=None  RotationAngleUnits=deg  RotationStandardAxis=+Z  RotationAngle=0.0  RotationArbitraryAxis=[0 0 1]  FollAlignAxisA=+X  BaseAlignAxisA=+Y  FollAlignAxisB=+Y  BaseAlignAxisB=+Z  RotationSequenceAxes=FollowerAxes  RotationSequence=XYX  RotationSequenceAngles=[0 0 0]  RotationSequenceAnglesUnits=deg  RotationMatrix=[1 0 0; 0 1 0; 0 0 1]
  Rigid Transform2 : sm_lib/Frames and Transforms/Rigid Transform  TranslationMethod=Cartesian  TranslationStandardOffset=0  TranslationLengthUnit=m  TranslationStandardAxis=+Z  TranslationCartesianOffset=[-d 0 0]  TranslationROffset=0  TranslationROffsetUnits=m  TranslationZOffset=0  TranslationZOffsetUnits=m  TranslationThetaOffset=0  TranslationThetaOffsetUnits=deg  RotationMethod=None  RotationAngleUnits=deg  RotationStandardAxis=+Z  RotationAngle=0.0  RotationArbitraryAxis=[0 0 1]  FollAlignAxisA=+X  BaseAlignAxisA=+Y  FollAlignAxisB=+Y  BaseAlignAxisB=+Z  RotationSequenceAxes=FollowerAxes  RotationSequence=XYX  RotationSequenceAngles=[0 0 0]  RotationSequenceAnglesUnits=deg  RotationMatrix=[1 0 0; 0 1 0; 0 0 1]
  Rigid Transform3 : sm_lib/Frames and Transforms/Rigid Transform  TranslationMethod=Cartesian  TranslationStandardOffset=0  TranslationLengthUnit=m  TranslationStandardAxis=+Z  TranslationCartesianOffset=[0 -d 0]  TranslationROffset=0  TranslationROffsetUnits=m  TranslationZOffset=0  TranslationZOffsetUnits=m  TranslationThetaOffset=0  TranslationThetaOffsetUnits=deg  RotationMethod=None  RotationAngleUnits=deg  RotationStandardAxis=+Z  RotationAngle=0.0  RotationArbitraryAxis=[0 0 1]  FollAlignAxisA=+X  BaseAlignAxisA=+Y  FollAlignAxisB=+Y  BaseAlignAxisB=+Z  RotationSequenceAxes=FollowerAxes  RotationSequence=XYX  RotationSequenceAngles=[0 0 0]  RotationSequenceAnglesUnits=deg  RotationMatrix=[1 0 0; 0 1 0; 0 0 1]
  Simscape Bus : SimscapeBus  HierarchyStrings=Marker1;Marker2;Marker3;Marker4
  Top : PMIOPort  Side=Left
  Geometry : PMIOPort  Port=2  Side=Right
  Markers : PMIOPort  Port=3  Side=Left
  connections:
  Brick Solid/LConn1 -- Top/RConn1 -- Rigid Transform3/LConn1 -- Rigid Transform2/LConn1 -- Rigid Transform1/LConn1 -- Rigid Transform/LConn1
  Brick Solid/RConn1 -- Geometry/RConn1
  Marker 1/LConn1 -- Rigid Transform/RConn1 -- Simscape Bus/LConn1
  Marker 2/LConn1 -- Simscape Bus/LConn2 -- Rigid Transform1/RConn1
  Marker 4/LConn1 -- Simscape Bus/LConn4 -- Rigid Transform3/RConn1
  Marker 3/LConn1 -- Simscape Bus/LConn3 -- Rigid Transform2/RConn1
  Markers/RConn1 -- Simscape Bus/RConn1

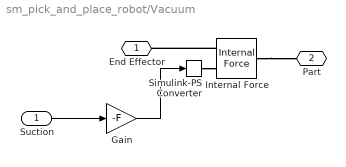
== system sm_pick_and_place_robot/Vacuum ==
  Suction : Inport
  Gain : Gain  Gain=-F
  Internal Force : sm_lib/Forces and Torques/Internal Force
      settings: SourceProductBaseCode=MS
  Simulink-PS Converter : nesl_utility/Simulink-PS Converter  PhysicalDomain=network_engine_domain  SubClassName=ps_input  LeftPortType=input  RightPortType=output  PseudoPeriodic=off  Frequencies=[]  NoiseDistribution=none  NoiseParameters=[]  Unit=N  AffineConversion=off  FilteringAndDerivatives=provide  SimscapeFilterOrder=1  InputFilterTimeConstant=0.001  UdotUserProvided=0
      settings: SourceProductBaseCode=PW,SS
  End Effector : PMIOPort  Side=Right
  Part : PMIOPort  Port=2  Side=Right
  wires:
  Gain/1 -> Simulink-PS Converter/1
  Suction/1 -> Gain/1
  connections:
  Simulink-PS Converter/RConn1 -- Internal Force/LConn2
  Internal Force/LConn1 -- End Effector/RConn1
  Internal Force/RConn1 -- Part/RConn1

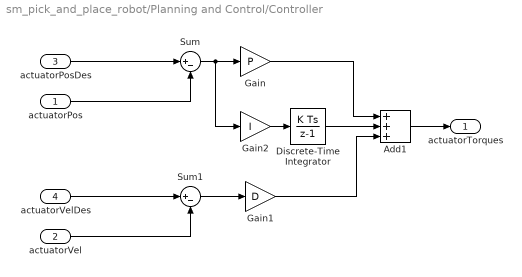
== system sm_pick_and_place_robot/Planning and Control/Controller ==
  actuatorPos : Inport
  actuatorVel : Inport  Port=2
  actuatorPosDes : Inport  Port=3
  actuatorVelDes : Inport  Port=4
  Add1 : Sum  Inputs=+++
  Discrete-Time Integrator : DiscreteIntegrator  gainval=1  SampleTime=-1  ICPrevOutput=DiscIntNeverNeededParam  ICPrevScaledInput=DiscIntNeverNeededParam
  Gain : Gain  Gain=P
  Gain1 : Gain  Gain=D
  Gain2 : Gain  Gain=I
  Sum : Sum  Inputs=|+-
  Sum1 : Sum  Inputs=|+-
  actuatorTorques : Outport
  wires:
  actuatorPosDes/1 -> Sum/1
  actuatorPos/1 -> Sum/2
  actuatorVel/1 -> Sum1/2
  Sum/1 -> Gain2/1, Gain/1
  Sum1/1 -> Gain1/1
  Gain/1 -> Add1/1
  Gain1/1 -> Add1/3
  Discrete-Time Integrator/1 -> Add1/2
  Gain2/1 -> Discrete-Time Integrator/1
  Add1/1 -> actuatorTorques/1
  actuatorVelDes/1 -> Sum1/1
